simulink model "mppt"  (R2024b)
settings: Solver=VariableStepAuto  StartTime=0.0  StopTime=Sim_Time  RelTol=1e-3
InitFcn:
  | run('../model_paramters/buck_converter_paramters.m')
undefined symbols (not defined in the file): Cin_calc, f_sw, L_calc, Lout, sampling, Sim_Time
libraries: spsSeriesRLCBranchLib x4, eeGeneralControl x3, spsCurrentMeasurementLib x2, simulink_extras x2, spsSampleandHoldLib x2, spsMosfetLib x2, spsVoltageMeasurementLib x2, spsDiodeLib x1, fuzblock x1, spsPVArrayLib x1, simulink x1, sps_lib x1
settings Model: LastModifiedBy=deso
settings DataIOCC: Decimation=60

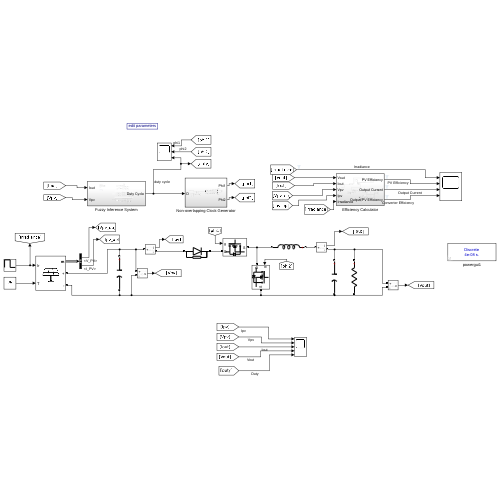
[thumbnail: Simulink's stored preview of the top-level diagram]
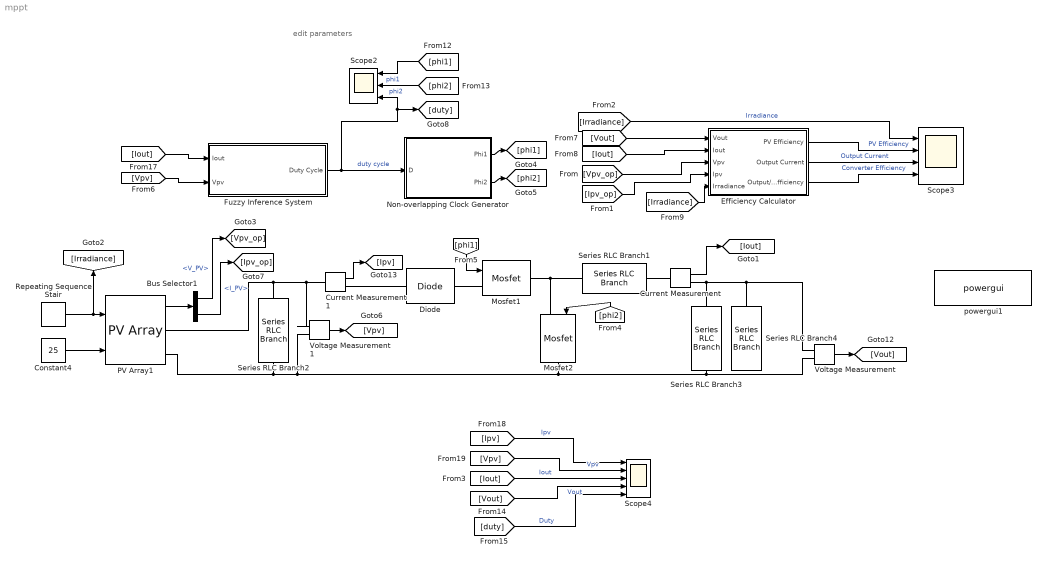
== system mppt ==
  note: edit parameters
  Bus Selector1 : BusSelector  OutputSignals=V_PV,I_PV
  Constant4 : Constant  Value=25
  Current Measurement : spsCurrentMeasurementLib/Current Measurement  PhasorSimulation=off  OutputType=Complex  PSBequivalent=0
  Current Measurement1 : spsCurrentMeasurementLib/Current Measurement  PhasorSimulation=off  OutputType=Complex  PSBequivalent=0
  Diode : spsDiodeLib/Diode  Ron=0.001  Lon=0  Vf=0.5  IC=0  UseSnubber=0  Rs=500  Cs=250e-9  Measurements=off
  Efficiency Calculator : Subsystem
  Fuzzy Inference System : Subsystem
  Mosfet1 : spsMosfetLib/Mosfet  Ron=10e-3  Lon=1e-9  Rd=0.01  Vfd=0.7  IC=0  Rs=1e5  Cs=inf  Measurements=off
  Mosfet2 : spsMosfetLib/Mosfet  Ron=10e-3  Lon=1e-9  Rd=0.01  Vfd=0.7  IC=0  Rs=1e5  Cs=inf  Measurements=off
  Non-overlapping Clock Generator : Subsystem
  PV Array1 : spsPVArrayLib/PV Array  Npar=1  Nser=1  PlotType=one module @ 25 deg.C & specified irradiances  S_vec="[ 1000  500  100 ]"  Temp_C_vec="[ 45 25  ]"  ModuleName=A10Green Technology A10J-M60-235  PlotWhenSelected=off  Pm=235.008  Ncell=60  Voc=36.72  Isc=8.23  Vm=30.6  Im=7.68  beta_Voc_pc=-0.359  alpha_Isc_pc=0.096999  beta_Voc=-0.13182  alpha_Isc=0.007983  IL=8.2383  I0=2.8335e-10  nI=0.98962  Rsh=196.9278  Rs=0.19811  RobustModel=off  RobustCellTemperature=313.3991  BAL=on  Tc=1e-6  Tfilter=5e-5
  Repeating Sequence Stair : simulink/Sources/Repeating Sequence Stair  OutValues=[1000 500].'  tsamp=Sim_Time*2/3  OutMin=[]  OutMax=[]  OutDataTypeStr=double  OutputDataTypeScalingMode=double  OutDataType=fixdt(0,8)  ConRadixGroup=Best Precision: Vector-wise  OutScaling=2^-12
  Scope2 : Scope  NumInputPorts=3
  Scope3 : Scope  NumInputPorts=4
  Scope4 : Scope  NumInputPorts=5
  Series RLC Branch1 : spsSeriesRLCBranchLib/Series RLC Branch  LConnTagsString=__new0  RConnTagsString=__new0  BranchType=L  Resistance=0  Inductance=L_calc  SetiL0=off  InitialCurrent=0  Capacitance=100e-6  Setx0=off  InitialVoltage=0  Measurements=None
  Series RLC Branch2 : spsSeriesRLCBranchLib/Series RLC Branch  LConnTagsString=__new0  RConnTagsString=__new0  BranchType=C  Resistance=0  Inductance=1e-6  SetiL0=off  InitialCurrent=0  Capacitance=Cin_calc  Setx0=off  InitialVoltage=0  Measurements=None
  Series RLC Branch3 : spsSeriesRLCBranchLib/Series RLC Branch  LConnTagsString=__new0  RConnTagsString=__new0  BranchType=C  Resistance=0  Inductance=Lout  SetiL0=off  InitialCurrent=0  Capacitance=2e3  Setx0=on  InitialVoltage=12  Measurements=None
  Series RLC Branch4 : spsSeriesRLCBranchLib/Series RLC Branch  LConnTagsString=__new0  RConnTagsString=__new0  BranchType=R  Resistance=10e3  Inductance=Lout  SetiL0=off  InitialCurrent=0  Capacitance=2e3  Setx0=on  InitialVoltage=12  Measurements=None
  Voltage Measurement : spsVoltageMeasurementLib/Voltage Measurement  PhasorSimulation=off  OutputType=Complex  PSBequivalent=0
  Voltage Measurement1 : spsVoltageMeasurementLib/Voltage Measurement  PhasorSimulation=off  OutputType=Complex  PSBequivalent=0
  powergui1 : sps_lib/powergui  Priority=1  SimulationMode=Discrete  SampleTime=1/(50*f_sw)  frequency=60  Iterations=50  frequencyindice=0  Pbase=100e6  ErrMax=1e-4  UnitsV=kV  UnitsW=MW  buscounter=0  FunctionMessages=off  echomessages=off  EnableUseOfTLC=off  CurrentSourceSwitches=off  DisableSnubberDevices=off  DisableRonSwitches=off  DisableVfSwitches=off  DisplayEquations=off  AutomaticDiscreteSolvers=off  SolverType=Tustin/Backward Euler (TBE)  Interpol=off  ExternalGateDelay=off  methode=off  Ts=100  x0status=blocks  SPID=on  SwTol=0  HookPort=off  NonlinearTolerance=1e-4  nMaxIteration=100  ContinueOnMaxIteration=off  RestoreLinks=warning  ResistiveCurrentMeasurement=off  Frange=[0:2:500]  Ylog=off  Xlog=on  ShowGrid=off  save=off  variable=ZData  structure=0  ZoomFFT=off  StartTime=0.0  cycles=1  DisplayStyle=1  fundamental=60  FreqAxis=off  MaxFrequency=1000  frequencyindicesteady=1  RmsSteady=1  display=off
  wires:
  Non-overlapping Clock Generator/2(Phi2) -> [phi2]
  [Vout] -> Efficiency Calculator/1(Vout)
  [Ipv_op] -> Efficiency Calculator/4(Ipv)
  [Iout] -> Efficiency Calculator/2(Iout)
  Non-overlapping Clock Generator/1(Phi1) -> [phi1]
  [Vpv_op] -> Efficiency Calculator/3(Vpv)
  Efficiency Calculator/3(Output/PV Efficiency) -> Scope3/4  "Converter Efficiency"
  Efficiency Calculator/1(PV Efficiency) -> Scope3/2  "PV Efficiency"
  PV Array1/1 -> Bus Selector1/1
  Efficiency Calculator/2(Output Current) -> Scope3/3  "Output Current"
  Constant4/1 -> PV Array1/2
  [Vpv] -> Fuzzy Inference System/2(Vpv)
  [Iout] -> Fuzzy Inference System/1(Iout)
  [phi2] -> Mosfet2/1
  [phi1] -> Mosfet1/1
  [Irradiance] -> Efficiency Calculator/5(Irradiance)
  [Irradiance] -> Scope3/1  "Irradiance"
  Fuzzy Inference System/1(Duty Cycle) -> Non-overlapping Clock Generator/1(D), [duty], Scope2/3  "duty cycle"
  [phi1] -> Scope2/1  "phi1"
  [phi2] -> Scope2/2  "phi2"
  Repeating Sequence Stair/1 -> [Irradiance], PV Array1/1
  [Vpv] -> Scope4/2  "Vpv"
  [Iout] -> Scope4/3  "Iout"
  [Vout] -> Scope4/4  "Vout"
  Voltage Measurement/1 -> [Vout]
  Current Measurement/1 -> [Iout]
  Voltage Measurement1/1 -> [Vpv]
  Current Measurement1/1 -> [Ipv]
  [duty] -> Scope4/5  "Duty"
  Bus Selector1/1 -> [Vpv_op]  "<V_PV>"
  Bus Selector1/2 -> [Ipv_op]  "<I_PV>"
  [Ipv] -> Scope4/1  "Ipv"
  connections:
  Voltage Measurement/LConn2 -- Series RLC Branch3/RConn1 -- Voltage Measurement1/LConn2 -- Series RLC Branch2/RConn1 -- PV Array1/RConn2 -- Mosfet2/RConn1
  Diode/RConn1 -- Mosfet1/LConn1
  Current Measurement1/LConn1 -- Voltage Measurement1/LConn1 -- Series RLC Branch2/LConn1 -- PV Array1/RConn1
  Mosfet1/RConn1 -- Series RLC Branch1/RConn1 -- Mosfet2/LConn1
  Current Measurement/RConn1 -- Series RLC Branch3/LConn1 -- Series RLC Branch4/LConn1 -- Voltage Measurement/LConn1
  Current Measurement1/RConn1 -- Diode/LConn1
  Series RLC Branch1/LConn1 -- Current Measurement/LConn1

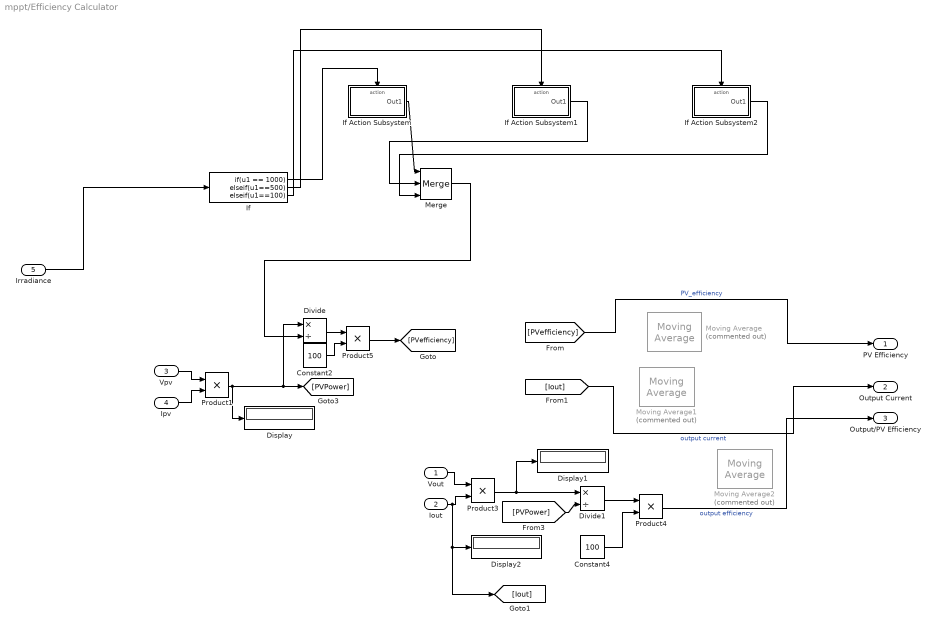
== system mppt/Efficiency Calculator ==
  Vout : Inport
  Iout : Inport  Port=2
  Vpv : Inport  Port=3
  Ipv : Inport  Port=4
  Irradiance : Inport  Port=5
  Constant2 : Constant  Value=100
  Constant4 : Constant  Value=100
  Display : Display
      settings: Format=decimal (Stored Integer)
  Display1 : Display
      settings: Format=decimal (Stored Integer)
  Display2 : Display
      settings: Format=decimal (Stored Integer)
  Divide : Product  Inputs=*/
  Divide1 : Product  Inputs=*/
  If : If  IfExpression=u1 == 1000  ElseIfExpressions=u1==500, u1==100  ShowElse=off
  If Action Subsystem : Subsystem  TreatAsAtomicUnit=on
  If Action Subsystem1 : Subsystem  TreatAsAtomicUnit=on
  If Action Subsystem2 : Subsystem  TreatAsAtomicUnit=on
  Merge : Merge  Inputs=3
  Moving Average : eeGeneralControl/Moving Average  Commented=on  VariantControl=Variant1  LabelModeActiveChoice=Discrete  f=100e3  x0=0  BufferSize=8192  Ts=-1
      settings: LibrarySourceBlock=ee_sl_lib/General Control/Moving Average
  Moving Average1 : eeGeneralControl/Moving Average  Commented=on  VariantControl=Variant1  LabelModeActiveChoice=Discrete  f=100e3  x0=0  BufferSize=8192  Ts=-1
      settings: LibrarySourceBlock=ee_sl_lib/General Control/Moving Average
  Moving Average2 : eeGeneralControl/Moving Average  Commented=on  VariantControl=Variant1  LabelModeActiveChoice=Discrete  f=100e3  x0=0  BufferSize=8192  Ts=-1
      settings: LibrarySourceBlock=ee_sl_lib/General Control/Moving Average
  Product{1,3..5} (4 alike) : Product
  PV Efficiency : Outport
  Output Current : Outport  Port=2
  Output/PV Efficiency : Outport  Port=3
  wires:
  Constant4/1 -> Product4/2
  Iout/1 -> [Iout], Display2/1, Product3/2
  Vout/1 -> Product3/1
  Divide1/1 -> Product4/1
  Product3/1 -> Display1/1, Divide1/1
  [PVPower] -> Divide1/2
  Product1/1 -> Divide/1, [PVPower], Display/1
  Vpv/1 -> Product1/1
  Ipv/1 -> Product1/2
  Irradiance/1 -> If/1
  Divide/1 -> Product5/1
  Constant2/1 -> Product5/2
  Product5/1 -> [PVefficiency]
  If/1 -> If Action Subsystem/Action
  If Action Subsystem/1(Out1) -> Merge/1
  If Action Subsystem1/1(Out1) -> Merge/2
  If Action Subsystem2/1(Out1) -> Merge/3
  Merge/1 -> Divide/2
  [Iout] -> Output Current/1  "output current"
  [PVefficiency] -> PV Efficiency/1  "PV_efficiency"
  Product4/1 -> Output/PV Efficiency/1  "output efficiency"
  If/2 -> If Action Subsystem1/Action
  If/3 -> If Action Subsystem2/Action

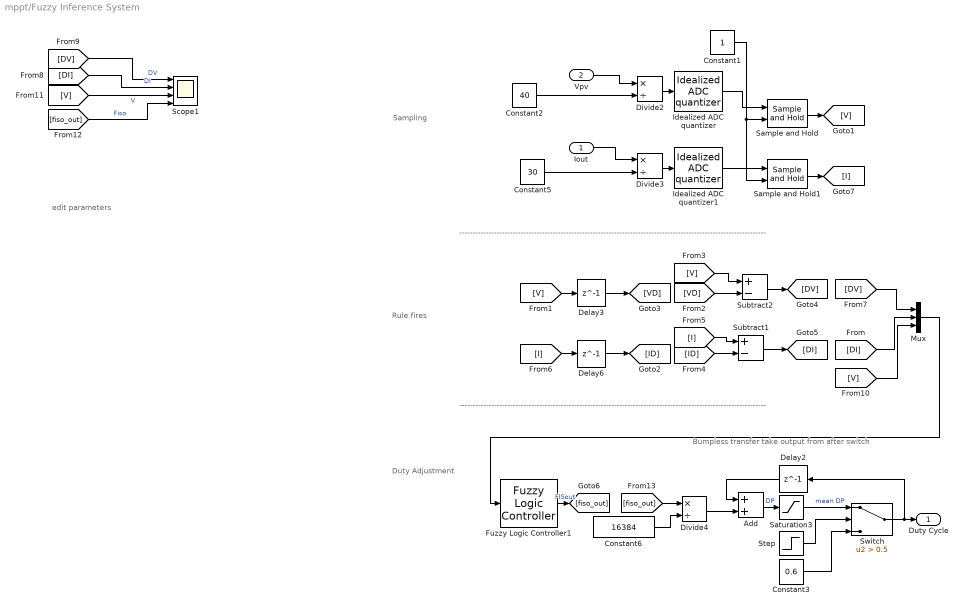
== system mppt/Fuzzy Inference System ==
  note: Bumpless transfer take output from after switch
  note: edit parameters
  note: -------------------------------------------------------------------------------------------------------------------
  note: -------------------------------------------------------------------------------------------------------------------
  note: Sampling
  note: Rule fires
  note: Duty Adjustment
  Iout : Inport
  Vpv : Inport  Port=2
  Add : Sum
  Constant1 : Constant
  Constant2 : Constant  Value=40
  Constant3 : Constant  Value=0.6
  Constant5 : Constant  Value=30
  Constant6 : Constant  Value=16384
  Delay2 : Delay  DelayLength=1  SampleTime=1/sampling
  Delay3 : Delay  DelayLength=1  SampleTime=1/sampling
  Delay6 : Delay  DelayLength=1  SampleTime=1/sampling
  Divide2 : Product  Inputs=*/
  Divide3 : Product  Inputs=*/
  Divide4 : Product  Inputs=*/
  Fuzzy Logic Controller1 : fuzblock/Fuzzy Logic  Controller  FIS='../fis_rules/mppt_sugeno.fis'  OutputSampleNumber=101  DataType=double  FuzzifiedInputs=off  RuleFiringStrengths=off  RuleOutputs=off  AggregatedOutputs=off  SimulateUsing=Interpreted execution  OutOfRangeInputValueMessage=warning  NoRuleFiredMessage=warning  EmptyOutputFuzzySetMessage=warning
  Idealized ADC quantizer : simulink_extras/Additional Discrete/Idealized ADC quantizer  NumberOfConverterBits=10  Vmin=0  Vmax=1  OutputDataType=int16  OutputNegativeValues=off
  Idealized ADC quantizer1 : simulink_extras/Additional Discrete/Idealized ADC quantizer  NumberOfConverterBits=10  Vmin=0  Vmax=1  OutputDataType=int16  OutputNegativeValues=off
  Mux : Mux  Inputs=3
  Sample and Hold : spsSampleandHoldLib/Sample and Hold  ic=0  Ts=1/sampling
      settings: LibrarySourceBlock=|
      | sps_lib/Control/Sample and
      | Hold
  Sample and Hold1 : spsSampleandHoldLib/Sample and Hold  ic=0  Ts=1/sampling
      settings: LibrarySourceBlock=|
      | sps_lib/Control/Sample and
      | Hold
  Saturation3 : Saturate  UpperLimit=0.75  LowerLimit=0.25
  Scope1 : Scope  NumInputPorts=4
  Step : Step  Time=Sim_Time/3
  Subtract1 : Sum  Inputs=+-
  Subtract2 : Sum  Inputs=+-
  Switch : Switch  Criteria=u2 > Threshold  Threshold=0.5  SaturateOnIntegerOverflow=off  InputSameDT=off
  Duty Cycle : Outport
  wires:
  Add/1 -> Saturation3/1  "DP"
  Saturation3/1 -> Switch/1  "mean DP"
  Delay2/1 -> Add/1
  Constant3/1 -> Switch/3
  Switch/1 -> Delay2/1, Duty Cycle/1
  Delay6/1 -> [ID]
  [ID] -> Subtract1/2
  [I] -> Delay6/1
  [V] -> Delay3/1
  [VD] -> Subtract2/2
  [V] -> Subtract2/1
  [DI] -> Mux/2
  [DV] -> Mux/1
  Mux/1 -> Fuzzy Logic Controller1/1
  [DI] -> Scope1/2  "DI"
  [DV] -> Scope1/1  "DV"
  Constant1/1 -> Sample and Hold1/2, Sample and Hold/2
  Idealized ADC quantizer/1 -> Sample and Hold/1
  Idealized ADC quantizer1/1 -> Sample and Hold1/1
  Sample and Hold/1 -> [V]
  Delay3/1 -> [VD]
  Divide2/1 -> Idealized ADC quantizer/1
  Vpv/1 -> Divide2/1
  Constant2/1 -> Divide2/2
  Iout/1 -> Divide3/1
  Divide3/1 -> Idealized ADC quantizer1/1
  Constant5/1 -> Divide3/2
  Divide4/1 -> Add/2
  Constant6/1 -> Divide4/2
  Step/1 -> Switch/2
  Sample and Hold1/1 -> [I]
  [I] -> Subtract1/1
  Fuzzy Logic Controller1/1 -> [fiso_out]  "FISout"
  [fiso_out] -> Scope1/4  "Fiso"
  [fiso_out] -> Divide4/1
  Subtract2/1 -> [DV]
  Subtract1/1 -> [DI]
  [V] -> Mux/3
  [V] -> Scope1/3  "V"

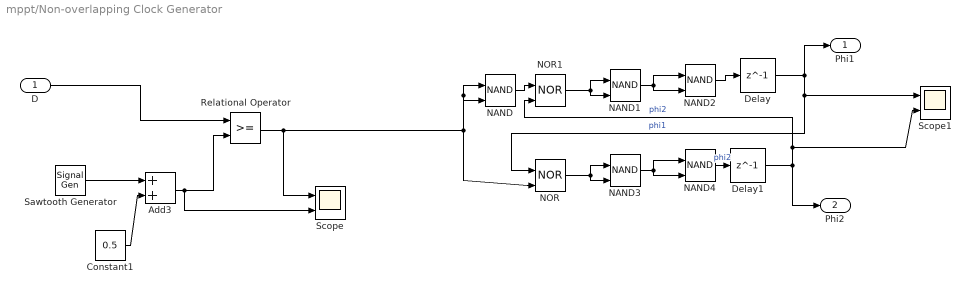
== system mppt/Non-overlapping Clock Generator ==
  D : Inport
  Add3 : Sum
  Constant1 : Constant  Value=0.5
  Delay : Delay  DelayLength=1  SampleTime=1/(f_sw*100)
  Delay1 : Delay  DelayLength=1  SampleTime=1/(f_sw*100)
  NAND{,1..4} (5 alike) : Logic  Operator=NAND  IconShape=distinctive  AllPortsSameDT=off  OutDataTypeStr=boolean
  NOR : Logic  Operator=NOR  IconShape=distinctive  AllPortsSameDT=off  OutDataTypeStr=boolean
  NOR1 : Logic  Operator=NOR  IconShape=distinctive  AllPortsSameDT=off  OutDataTypeStr=boolean
  Relational Operator : RelationalOperator  OutDataTypeStr=boolean  RndMeth=Simplest  InputSameDT=off
  Sawtooth Generator : SignalGenerator  WaveForm=sawtooth  Amplitude=-0.5  Frequency=f_sw
  Scope : Scope  NumInputPorts=2
  Scope1 : Scope  NumInputPorts=2
  Phi1 : Outport
  Phi2 : Outport  Port=2
  wires:
  NOR/1 -> NAND3/1, NAND3/2
  NAND3/1 -> NAND4/1, NAND4/2
  NAND/1 -> NOR1/1
  NOR1/1 -> NAND1/1, NAND1/2
  Delay1/1 -> NOR1/2, Scope1/2, Phi2/1  "phi2"
  NAND2/1 -> Delay/1
  Delay/1 -> NOR/1, Scope1/1, Phi1/1  "phi1"
  NAND1/1 -> NAND2/1, NAND2/2
  Relational Operator/1 -> NOR/2, NAND/2, NAND/1, Scope/1
  Constant1/1 -> Add3/2
  Sawtooth Generator/1 -> Add3/1
  Add3/1 -> Scope/2, Relational Operator/2
  D/1 -> Relational Operator/1
  NAND4/1 -> Delay1/1  "phi2"

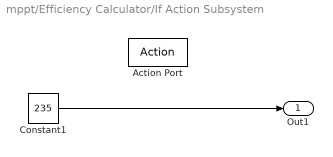
== system mppt/Efficiency Calculator/If Action Subsystem ==
  Action Port : ActionPort  ActionPortLabel=if(u1 == 1000)
  Constant1 : Constant  Value=235
  Out1 : Outport
  wires:
  Constant1/1 -> Out1/1

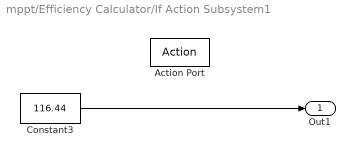
== system mppt/Efficiency Calculator/If Action Subsystem1 ==
  Action Port : ActionPort  ActionPortLabel=elseif(u1==500)
  Constant3 : Constant  Value=116.44
  Out1 : Outport
  wires:
  Constant3/1 -> Out1/1

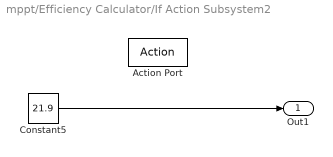
== system mppt/Efficiency Calculator/If Action Subsystem2 ==
  Action Port : ActionPort  ActionPortLabel=elseif( u1==100)
  Constant5 : Constant  Value=21.9
  Out1 : Outport
  wires:
  Constant5/1 -> Out1/1
